simulink model "HybridControllerD2D2sim"  (R2019a)
settings: Solver=FixedStepDiscrete  StartTime=0.0  StopTime=inf  FixedStep=controlPeriod  RelTol=1e-3
PreLoadFcn:
  | initializeSimulation
  | initializeSCRAMNetGT
values from neighbouring files (symbols this model uses):
  controlPeriod = 1/1024    (= 0.0009765625)    [initializeSimulation.m]
undefined symbols (not defined in the file or in its folder): HybridCtrlParameters
libraries: simulink x4, HybridSimLib x1, slrtlib x1
settings Model: ExtModeArmWhenConnect=off  Creator=Andreas Schellenberg  LastModifiedBy=Andreas
settings DataIOCC: SaveFormat=Array  SaveOutput=off  SignalLogging=off  SaveTime=off  ReturnWorkspaceOutputs=off  SignalLoggingName=sigsOut
settings OptimizationCC: BlockReduction=off  OptimizeBlockIOStorage=off  BufferReuse=off  GlobalBufferReuse=off  ExpressionFolding=off  ExpressionDepthLimit=2147483647  LocalBlockOutputs=off  InitFltsAndDblsToZero=on  EfficientFloat2IntCast=on  LifeSpan=inf  SimCompilerOptimization=on  OptimizeDataStoreBuffers=off  BusAssignmentInplaceUpdate=off
settings DebuggingCC: SaveWithParameterizedLinksMsg=none  CheckSSInitialOutputMsg=off  UnderspecifiedInitializationDetection=Classic  StateNameClashWarn=warning  SFUnexpectedBacktrackingDiag=warning  SFNoUnconditionalDefaultTransitionDiag=warning  SFExecutionAtInitializationDiag=none  ArithmeticOperatorsInVariantConditions=warning
settings HardwareCC: ProdBitPerPointer=32  ProdBitPerSizeT=32  ProdBitPerPtrDiffT=32  ProdLargestAtomicFloat=None  ProdWordSize=32  ProdLongLongMode=on  ProdHWDeviceType=Generic->32-bit x86 compatible  TargetIntDivRoundTo=Zero  TargetEndianess=LittleEndian  TargetHWDeviceType=Intel->x86/Pentium
settings ModelReferenceCC: PropagateSignalLabelsOutOfModel=off
settings SFSimCC: SimCustomHeaderCode="#include \"PredictorCorrector.h\""  SimUserSources=PredictorCorrector.c  SimUserIncludeDirs="\"C:\\Program Files\\OpenFresco\\SourceCode\\SRC\\experimentalControl\\Simulink\\HybridSimToolbox\""  SimUseLocalCustomCode=off  SimParseCustomCode=off
settings RTWCC: SystemTargetFile=slrt.tlc  TemplateMakefile=slrt_default_tmf  Description=Simulink Real-Time  RTWUseLocalCustomCode=off  CustomHeaderCode="#include \"PredictorCorrector.h\""  CustomInclude="\"C:\\Program Files\\OpenFresco\\SourceCode\\SRC\\experimentalControl\\Simulink\\HybridSimToolbox\""  CustomSource=PredictorCorrector.c  CodeExecutionProfiling=on  RTWCompilerOptimization=on
settings CodeAppCC: StateflowObjectComments=on
settings SimulinkRealTimeCC: TargetFcnLib=ansi_tfl_tmw.mat  GeneratePreprocessorConditionals=Disable all  PreserveStateflowLocalDataDimensions=off
settings ConfigComp: CovMetricSettings=dw  CovHtmlReporting=on  CovSaveCumulativeToWorkspaceVar=on  CovSaveSingleToWorkspaceVar=on  CovExternalEMLEnable=off  CovSFcnEnable=off

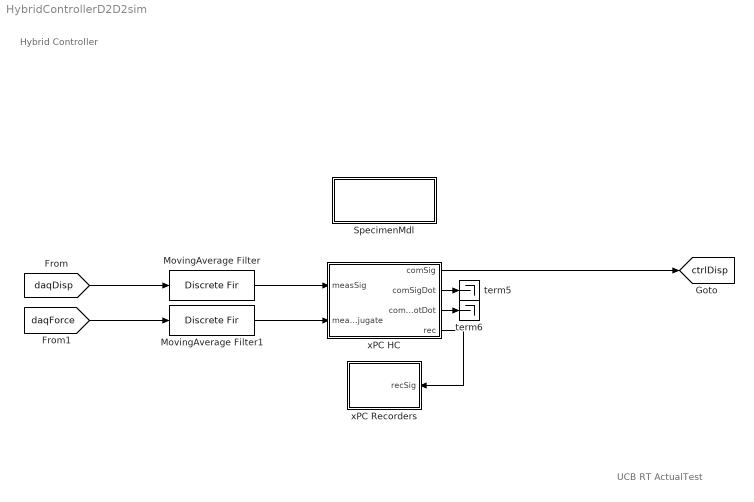
== system HybridControllerD2D2sim ==
  note: Hybrid Controller
  note: UCB RT ActualTest
  MovingAverage Filter : DiscreteFir  Coefficients=1/numSample*ones(1,numSample)  mask(Moving Average Filter){numSample=1}
      mask prompts: numSample "Number of Samples: numSample"
      mask help:
      | Moving average filter by using discrete FIR filter.
      | Set numSample = 1 for no filtering.
      mask Display: fprintf('MovingAverage\nFilter')
  MovingAverage Filter1 : DiscreteFir  Coefficients=1/numSample*ones(1,numSample)  mask(Moving Average Filter){numSample=1}
      mask prompts: numSample "Number of Samples: numSample"
      mask help:
      | Moving average filter by using discrete FIR filter.
      | Set numSample = 1 for no filtering.
      mask Display: fprintf('MovingAverage\nFilter')
  SpecimenMdl : Subsystem
      mask Display: fprintf('Test\nSpecimen');
  term5 : Terminator
  term6 : Terminator
  xPC HC : Subsystem  mask(Hybrid Controller: D2/D2){hcp=HybridCtrlParameters, node=struct([])}
      mask prompts: hcp "Hybrid control parameter structure"; node "SCRAMNet node structure"
      mask help: Hybrid Controller using C0-continuous quadratic Lagrange interpolation for prediction and correction
      mask init:
      | if isfield(hcp,'nDOF')
      |     nDOF = hcp.nDOF;
      | else
      |     nDOF = 1;
      | end
      | if isfield(hcp,'upFact')
      |     upFact = hcp.upFact;
      | else
      |     upFact = 1;
      | end
      | if isfield(hcp,'iDelay')
      |     iDelay = hcp.iDelay;
      | else
      |     iDelay = zeros(nDOF);
      | end
      | dtInt = hcp.dtInt;
      | dtSim = hcp.dtSim;
      | dtCon = hcp.dtCon;
      | N = hcp.N;
      mask Display: disp('xPC Target\nHybrid Controller\n(D2/D2)')
  xPC Recorders : Subsystem  mask{nDOF=HybridCtrlParameters.nDOF}
      mask prompts: nDOF "Number of DOF: nDOF"
  tag scope: ctrlDisp=global
  wires:
  [daqDisp] -> MovingAverage Filter/1
  xPC HC/1(comSig) -> [ctrlDisp]
  [daqForce] -> MovingAverage Filter1/1
  xPC HC/2(comSigDot) -> term5/1
  xPC HC/3(comSigDotDot) -> term6/1
  xPC HC/4(rec) -> xPC Recorders/1(recSig)
  MovingAverage Filter/1 -> xPC HC/1(measSig)
  MovingAverage Filter1/1 -> xPC HC/2(measSigConjugate)

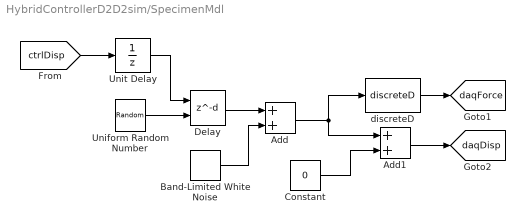
== system HybridControllerD2D2sim/SpecimenMdl ==
  Add : Sum
  Add1 : Sum
  Band-Limited White Noise : simulink/Sources/Band-Limited White Noise  Cov=1e-7  Ts=controlPeriod  seed=[23341]
  Constant : Constant  Value=0
  Delay : Delay  DelayLengthSource=Input port  DelayLengthUpperLimit=20
      settings: InputPortMap=u0,p1
  Uniform Random Number : UniformRandomNumber  Minimum=0  Maximum=2  SampleTime=controlPeriod
  Unit Delay : UnitDelay  SampleTime=-1  HasFrameUpgradeWarning=on
  discreteD : HybridSimLib/Material Models/discreteD  k=2.8  fy=1.5  alpha=0.01  beta=0.5  gamma=0.5  n=2  dt=controlPeriod
      settings: SourceProductName=Hybrid Simulation
  tag scope: daqDisp=global, daqForce=global
  wires:
  discreteD/1 -> [daqForce]
  Add/1 -> Add1/1, discreteD/1
  Delay/1 -> Add/1
  Band-Limited White Noise/1 -> Add/2
  Uniform Random Number/1 -> Delay/2
  [ctrlDisp] -> Unit Delay/1
  Unit Delay/1 -> Delay/1
  Add1/1 -> [daqDisp]
  Constant/1 -> Add1/2

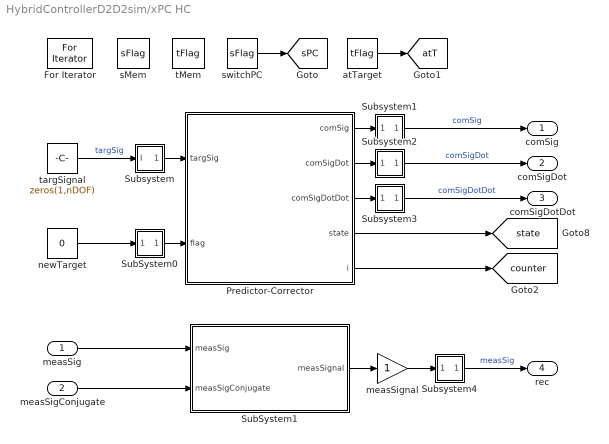
== system HybridControllerD2D2sim/xPC HC ==
  measSig : Inport
  measSigConjugate : Inport  Port=2
  For Iterator : ForIterator  IterationLimit=upFact  ShowIterationPort=off
  Predictor-Corrector : Stateflow chart  TreatAsAtomicUnit=on
  SubSystem0 : Subsystem
      mask Display: disp('I/O')
  SubSystem1 : Subsystem
  Subsystem : Subsystem
      mask Display: disp('I/O')
  Subsystem1 : Subsystem
      mask Display: disp('I/O')
  Subsystem2 : Subsystem
      mask Display: disp('I/O')
  Subsystem3 : Subsystem
      mask Display: disp('I/O')
  Subsystem4 : Subsystem
      mask Display: disp('I/O')
  atTarget : DataStoreRead  DataStoreName=tFlag
  measSignal : Gain  OutDataTypeStr=double
  newTarget : Constant  Value=0  OutDataTypeStr=int32  SampleTime=-1
  sMem : DataStoreMemory  DataStoreName=sFlag  ShowAdditionalParam=off  OutDataTypeStr=int32
  switchPC : DataStoreRead  DataStoreName=sFlag
  tMem : DataStoreMemory  DataStoreName=tFlag  ShowAdditionalParam=off  OutDataTypeStr=int32
  targSignal : Constant  Value=zeros(1,nDOF)  OutDataTypeStr=double  SampleTime=-1
  comSig : Outport
  comSigDot : Outport  Port=2
  comSigDotDot : Outport  Port=3
  rec : Outport  Port=4
  tag scope: atT=global, counter=global, sPC=global, state=global
  wires:
  measSignal/1 -> Subsystem4/1(measSig)
  SubSystem1/1(measSignal) -> measSignal/1
  Predictor-Corrector/5(i) -> [counter]
  SubSystem0/1(Out) -> Predictor-Corrector/2(flag)
  switchPC/1 -> [sPC]
  atTarget/1 -> [atT]
  targSignal/1 -> Subsystem/1(I)  "targSig"
  Subsystem/1(O) -> Predictor-Corrector/1(targSig)
  measSig/1 -> SubSystem1/1(measSig)
  measSigConjugate/1 -> SubSystem1/2(measSigConjugate)
  Predictor-Corrector/1(comSig) -> Subsystem1/1(In)
  Predictor-Corrector/2(comSigDot) -> Subsystem2/1(In)
  Predictor-Corrector/3(comSigDotDot) -> Subsystem3/1(In)
  newTarget/1 -> SubSystem0/1(In)
  Predictor-Corrector/4(state) -> [state]
  Subsystem2/1(Out) -> comSigDot/1  "comSigDot"
  Subsystem3/1(Out) -> comSigDotDot/1  "comSigDotDot"
  Subsystem1/1(Out) -> comSig/1  "comSig"
  Subsystem4/1(Out1) -> rec/1  "measSig"

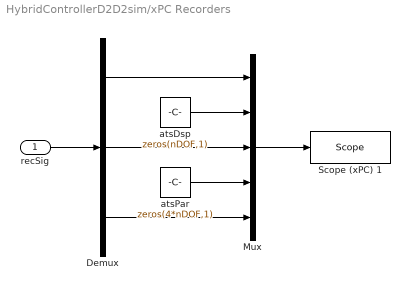
== system HybridControllerD2D2sim/xPC Recorders ==
  recSig : Inport
  Demux : Demux  Outputs=[(4*nDOF) (4*nDOF) 5]
  Mux : Mux  Inputs=5
  Scope (xPC) 1 : slrtlib/Displays and Logging/Scope   scopeno=1  scopetype=File  autostart=on  viewmode=Numerical  formatstr='%15.6f'  grid=on  ylimits=[-4,4]  nosamples=60*1024  noprepostsamples=0  interleave=1  triggermode=FreeRun  triggersignal=1  trigsignalfromport=off  triggerlevel=0.0  triggerslope=Either  triggerscope=1  triggersample=0  filename=H:\xpcRec.dat  mode=Lazy  writesize=512  autorestart=on  dynamicfilemode=off  maxwritefilesize=512*1024^2
  atsDsp : Constant  Value=zeros(nDOF,1)
  atsPar : Constant  Value=zeros(4*nDOF,1)
  wires:
  recSig/1 -> Demux/1
  atsDsp/1 -> Mux/2
  atsPar/1 -> Mux/4
  Demux/1 -> Mux/1
  Demux/2 -> Mux/3
  Mux/1 -> Scope (xPC) 1/1
  Demux/3 -> Mux/5

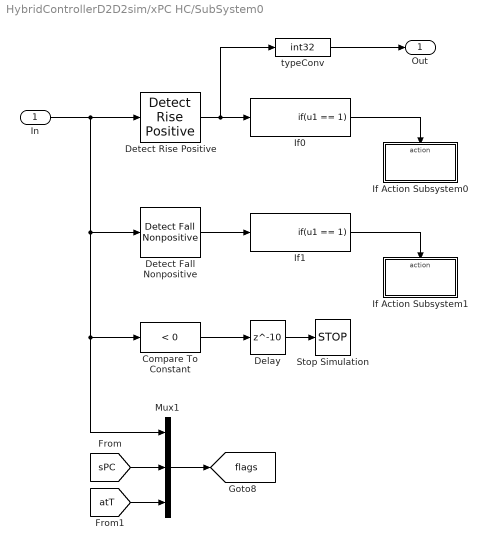
== system HybridControllerD2D2sim/xPC HC/SubSystem0 ==
  In : Inport
  Compare To Constant : simulink/Logic and Bit Operations/Compare To Constant  relop=<  const=0  OutDataTypeStr=boolean
  Delay : Delay  DelayLength=10
  Detect Fall Nonpositive : simulink/Logic and Bit Operations/Detect Fall Nonpositive  vinit=0  OutDataTypeStr=uint8
      settings: SourceProductName=Simulink  SourceProductBaseCode=SL
  Detect Rise Positive : simulink/Logic and Bit Operations/Detect Rise Positive  vinit=0  OutDataTypeStr=uint8
  If Action Subsystem0 : Subsystem  TreatAsAtomicUnit=on
  If Action Subsystem1 : Subsystem  TreatAsAtomicUnit=on
  If0 : If  IfExpression=u1 == 1  ShowElse=off
  If1 : If  IfExpression=u1 == 1  ShowElse=off
  Mux1 : Mux  Inputs=3
  Stop Simulation : Stop
  typeConv : DataTypeConversion  OutDataTypeStr=int32  SaturateOnIntegerOverflow=on  RndMeth=Zero
  Out : Outport
  tag scope: flags=global
  wires:
  Detect Rise Positive/1 -> If0/1, typeConv/1
  Detect Fall Nonpositive/1 -> If1/1
  If1/1 -> If Action Subsystem1/Action
  If0/1 -> If Action Subsystem0/Action
  typeConv/1 -> Out/1
  Mux1/1 -> [flags]
  [sPC] -> Mux1/2
  [atT] -> Mux1/3
  In/1 -> Detect Rise Positive/1, Detect Fall Nonpositive/1, Compare To Constant/1, Mux1/1
  Compare To Constant/1 -> Delay/1
  Delay/1 -> Stop Simulation/1

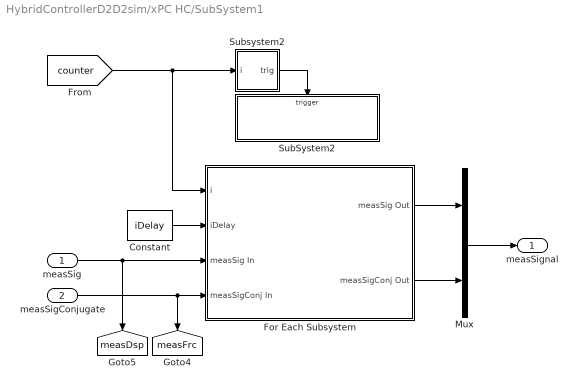
== system HybridControllerD2D2sim/xPC HC/SubSystem1 ==
  measSig : Inport
  measSigConjugate : Inport  Port=2
  Constant : Constant  Value=iDelay
  For Each Subsystem : Subsystem  TreatAsAtomicUnit=on
  Mux : Mux  Inputs=2
  SubSystem2 : Subsystem  TreatAsAtomicUnit=on
  Subsystem2 : Subsystem
  measSignal : Outport
  tag scope: measDsp=global, measFrc=global
  wires:
  Subsystem2/1(trig) -> SubSystem2/Trigger
  [counter] -> Subsystem2/1(i), For Each Subsystem/1(i)
  Constant/1 -> For Each Subsystem/2(iDelay)
  measSig/1 -> For Each Subsystem/3(measSig In), [measDsp]
  measSigConjugate/1 -> For Each Subsystem/4(measSigConj In), [measFrc]
  For Each Subsystem/1(measSig Out) -> Mux/1
  For Each Subsystem/2(measSigConj Out) -> Mux/2
  Mux/1 -> measSignal/1

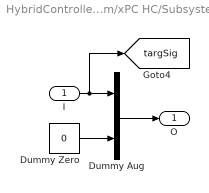
== system HybridControllerD2D2sim/xPC HC/Subsystem ==
  I : Inport  PortDimensions=nDOF
  Dummy Aug : Mux  Inputs=[nDOF 1]
  Dummy Zero : Constant  Value=0  OutDataTypeStr=double  SampleTime=-1
  O : Outport  PortDimensions=nDOF+1
  tag scope: targSig=global
  wires:
  Dummy Zero/1 -> Dummy Aug/2
  I/1 -> Dummy Aug/1, [targSig]
  Dummy Aug/1 -> O/1

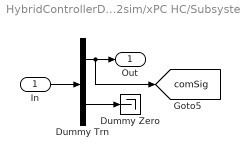
== system HybridControllerD2D2sim/xPC HC/Subsystem1 ==
  In : Inport  PortDimensions=nDOF+1
  Dummy Trn : Demux  Outputs=[nDOF 1]
  Dummy Zero : Terminator
  Out : Outport  PortDimensions=nDOF
  tag scope: comSig=global
  wires:
  Dummy Trn/2 -> Dummy Zero/1
  Dummy Trn/1 -> Out/1, [comSig]
  In/1 -> Dummy Trn/1

== system HybridControllerD2D2sim/xPC HC/Subsystem2 ==
  In : Inport  PortDimensions=nDOF+1
  Dummy Trn : Demux  Outputs=[nDOF 1]
  Dummy Zero : Terminator
  Out : Outport  PortDimensions=nDOF
  tag scope: comSigDot=global
  wires:
  Dummy Trn/2 -> Dummy Zero/1
  Dummy Trn/1 -> Out/1, [comSigDot]
  In/1 -> Dummy Trn/1

== system HybridControllerD2D2sim/xPC HC/Subsystem3 ==
  In : Inport  PortDimensions=nDOF+1
  Dummy Trn : Demux  Outputs=[nDOF 1]
  Dummy Zero : Terminator
  Out : Outport  PortDimensions=nDOF
  tag scope: comSigDotDot=global
  wires:
  Dummy Trn/2 -> Dummy Zero/1
  Dummy Trn/1 -> Out/1, [comSigDotDot]
  In/1 -> Dummy Trn/1

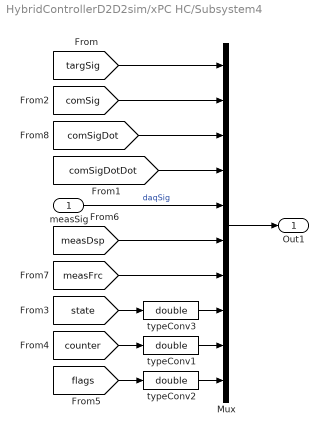
== system HybridControllerD2D2sim/xPC HC/Subsystem4 ==
  measSig : Inport
  Mux : Mux  Inputs=10
  typeConv1 : DataTypeConversion  OutDataTypeStr=double  SaturateOnIntegerOverflow=on  RndMeth=Zero
  typeConv2 : DataTypeConversion  OutDataTypeStr=double  SaturateOnIntegerOverflow=on  RndMeth=Zero
  typeConv3 : DataTypeConversion  OutDataTypeStr=double  SaturateOnIntegerOverflow=on  RndMeth=Zero
  Out1 : Outport
  wires:
  measSig/1 -> Mux/5  "daqSig"
  [flags] -> typeConv2/1
  [counter] -> typeConv1/1
  [state] -> typeConv3/1
  typeConv3/1 -> Mux/8
  typeConv1/1 -> Mux/9
  typeConv2/1 -> Mux/10
  [measFrc] -> Mux/7
  [measDsp] -> Mux/6
  [comSigDotDot] -> Mux/4
  [comSigDot] -> Mux/3
  [comSig] -> Mux/2
  [targSig] -> Mux/1
  Mux/1 -> Out1/1

== system HybridControllerD2D2sim/xPC HC/SubSystem0/If Action Subsystem0 ==
  Action Port : ActionPort  PropagateVarSize=During execution  ActionPortLabel=if(u1 == 1)
  Data Store Write0 : DataStoreWrite  DataStoreName=sFlag
  Data Store Write1 : DataStoreWrite  DataStoreName=tFlag
  atTargetFlag : Constant  Value=0  OutDataTypeStr=int32  SampleTime=-1
  switchFlag : Constant  OutDataTypeStr=int32  SampleTime=-1
  wires:
  atTargetFlag/1 -> Data Store Write1/1
  switchFlag/1 -> Data Store Write0/1

== system HybridControllerD2D2sim/xPC HC/SubSystem0/If Action Subsystem1 ==
  Action Port : ActionPort  PropagateVarSize=During execution  ActionPortLabel=if(u1 == 1)
  Data Store Write0 : DataStoreWrite  DataStoreName=sFlag
  switchFlag : Constant  Value=0  OutDataTypeStr=int32  SampleTime=-1
  wires:
  switchFlag/1 -> Data Store Write0/1

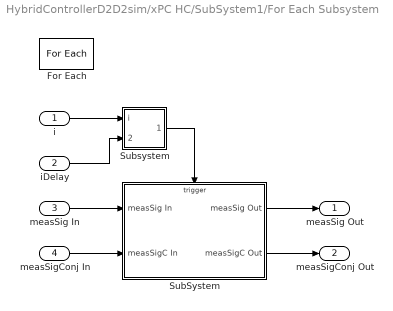
== system HybridControllerD2D2sim/xPC HC/SubSystem1/For Each Subsystem ==
  i : Inport
  iDelay : Inport  Port=2  Partition=on  PartitionDimension=1  PartitionWidth=1  PartitionOffset=0
  measSig In : Inport  Port=3  Partition=on  PartitionDimension=1  PartitionWidth=1  PartitionOffset=0
  measSigConj In : Inport  Port=4  Partition=on  PartitionDimension=1  PartitionWidth=1  PartitionOffset=0
  For Each : ForEach  DisableCoverage=on  IndexMode=One-based
  SubSystem : Subsystem  TreatAsAtomicUnit=on
  Subsystem : Subsystem
  measSig Out : Outport  ConcatenationDimension=1
  measSigConj Out : Outport  Port=2  ConcatenationDimension=1
  wires:
  Subsystem/1(trig) -> SubSystem/Trigger
  measSig In/1 -> SubSystem/1(measSig In)
  measSigConj In/1 -> SubSystem/2(measSigC In)
  SubSystem/1(measSig Out) -> measSig Out/1
  SubSystem/2(measSigC Out) -> measSigConj Out/1
  iDelay/1 -> Subsystem/2(iDelay)
  i/1 -> Subsystem/1(i)

== system HybridControllerD2D2sim/xPC HC/SubSystem1/SubSystem2 ==
  Trigger : TriggerPort  VariantControl=(inherit)
  Data Store Write : DataStoreWrite  DataStoreName=tFlag
  atTargetFlag : Constant  OutDataTypeStr=int32  SampleTime=-1
  wires:
  atTargetFlag/1 -> Data Store Write/1

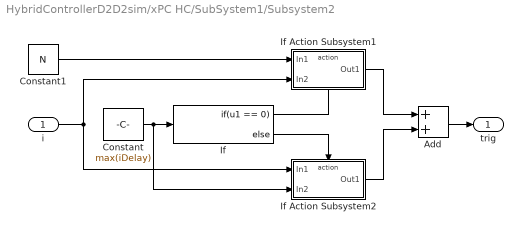
== system HybridControllerD2D2sim/xPC HC/SubSystem1/Subsystem2 ==
  i : Inport
  Add : Sum
  Constant : Constant  Value=max(iDelay)
  Constant1 : Constant  Value=N
  If : If  IfExpression=u1 == 0
  If Action Subsystem1 : Subsystem  TreatAsAtomicUnit=on
  If Action Subsystem2 : Subsystem  TreatAsAtomicUnit=on
  trig : Outport
  wires:
  Constant/1 -> If/1, If Action Subsystem2/2(In2)
  If/1 -> If Action Subsystem1/Action
  If/2 -> If Action Subsystem2/Action
  If Action Subsystem1/1(Out1) -> Add/1
  If Action Subsystem2/1(Out1) -> Add/2
  Add/1 -> trig/1
  i/1 -> If Action Subsystem1/2(In2), If Action Subsystem2/1(In1)
  Constant1/1 -> If Action Subsystem1/1(In1)

== system HybridControllerD2D2sim/xPC HC/SubSystem1/For Each Subsystem/SubSystem ==
  measSig In : Inport
  measSigC In : Inport  Port=2
  Trigger : TriggerPort  VariantControl=(inherit)
  measSig Out : Outport  InitialOutput=[0]
  measSigC Out : Outport  Port=2  InitialOutput=[0]
  wires:
  measSigC In/1 -> measSigC Out/1
  measSig In/1 -> measSig Out/1

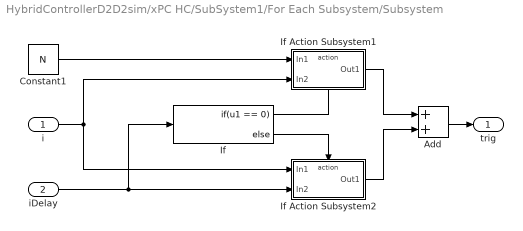
== system HybridControllerD2D2sim/xPC HC/SubSystem1/For Each Subsystem/Subsystem ==
  i : Inport
  iDelay : Inport  Port=2
  Add : Sum
  Constant1 : Constant  Value=N
  If : If  IfExpression=u1 == 0
  If Action Subsystem1 : Subsystem  TreatAsAtomicUnit=on
  If Action Subsystem2 : Subsystem  TreatAsAtomicUnit=on
  trig : Outport
  wires:
  iDelay/1 -> If/1, If Action Subsystem2/2(In2)
  If/1 -> If Action Subsystem1/Action
  If/2 -> If Action Subsystem2/Action
  If Action Subsystem1/1(Out1) -> Add/1
  If Action Subsystem2/1(Out1) -> Add/2
  Add/1 -> trig/1
  i/1 -> If Action Subsystem1/2(In2), If Action Subsystem2/1(In1)
  Constant1/1 -> If Action Subsystem1/1(In1)

== system HybridControllerD2D2sim/xPC HC/SubSystem1/Subsystem2/If Action Subsystem1 ==
  In1 : Inport
  In2 : Inport  Port=2
  Action Port : ActionPort  ActionPortLabel=if(u1 == 0)
  Relational Operator : RelationalOperator  Operator===  OutDataTypeStr=boolean  RndMeth=Nearest
  Out1 : Outport  InitialOutput=0
  wires:
  Relational Operator/1 -> Out1/1
  In1/1 -> Relational Operator/1
  In2/1 -> Relational Operator/2

== system HybridControllerD2D2sim/xPC HC/SubSystem1/Subsystem2/If Action Subsystem2 ==
  In1 : Inport
  In2 : Inport  Port=2
  Action Port : ActionPort  ActionPortLabel=else
  Relational Operator : RelationalOperator  Operator===  OutDataTypeStr=boolean  RndMeth=Nearest
  Out1 : Outport  InitialOutput=0
  wires:
  Relational Operator/1 -> Out1/1
  In1/1 -> Relational Operator/1
  In2/1 -> Relational Operator/2

== system HybridControllerD2D2sim/xPC HC/SubSystem1/For Each Subsystem/Subsystem/If Action Subsystem1 ==
  In1 : Inport
  In2 : Inport  Port=2
  Action Port : ActionPort  ActionPortLabel=if(u1 == 0)
  Relational Operator : RelationalOperator  Operator===  OutDataTypeStr=boolean  RndMeth=Nearest
  Out1 : Outport  InitialOutput=0
  wires:
  Relational Operator/1 -> Out1/1
  In1/1 -> Relational Operator/1
  In2/1 -> Relational Operator/2

== system HybridControllerD2D2sim/xPC HC/SubSystem1/For Each Subsystem/Subsystem/If Action Subsystem2 ==
  In1 : Inport
  In2 : Inport  Port=2
  Action Port : ActionPort  ActionPortLabel=else
  Relational Operator : RelationalOperator  Operator===  OutDataTypeStr=boolean  RndMeth=Nearest
  Out1 : Outport  InitialOutput=0
  wires:
  Relational Operator/1 -> Out1/1
  In1/1 -> Relational Operator/1
  In2/1 -> Relational Operator/2

== stateflow chart HybridControllerD2D2sim/xPC HC/Predictor-Corrector ==
  state HybridController [parallel]
    settings: executionOrder=1
    state Initialize
      en:
      state = -1;
      i = 0; iSD = 0; diSD = 1;
      initData(nDOF,dtCon,dtSim,dtInt);
      state GetSetpoint
        en:
        setData(targSig);
        setSig(comSig,targSig);
        zeroSig(comSigDot);
        zeroSig(comSigDotDot);
        du:
        i = 0;
      (default) -> GetSetpoint
      GetSetpoint -> GetSetpoint : [after(dtCon,sec)]
          | {i=N}
    state Correct
      en:
      state = 0;
      setCurSig(comSig,i/N);
      setNewSig(targSig);
      en, du:
      di = min(max(diSD+1/(0.1*N)*(i-iSD),0.001),1.0);
      i = min(i+di,N);
      correctD2(comSig,i/N);
      correctV2(comSigDot,i/N);
      correctA2(comSigDotDot,i/N);
    state Predict
      en:
      state = 1;
      setCurSig(comSig,1.0);
      i = 1; iSD = 0; diSD = 1;
      du:
      i++;
      en, du:
      predictD2(comSig,i/N);
      predictV2(comSigDot,i/N);
      predictA2(comSigDotDot,i/N);
    state AutoSlowDown
      en:
      state = 2;
      en, du:
      diSD = 9-i/(0.1*N); i += diSD; iSD = i;
      predictD2(comSig,i/N);
      predictV2(comSigDot,i/N);
      predictA2(comSigDotDot,i/N);
    Correct -> Predict [order 1] : [flag==0 && i==N]
    (default) -> Initialize
    Initialize -> Correct : [flag==1]
        | {i=0}
    Predict -> Correct [order 2] : [flag==1]
    Predict -> AutoSlowDown [order 1] : [flag==0 && i>=0.8*N]
    AutoSlowDown -> Correct : [flag==1]
    Correct -> Correct [order 2] : [flag==1]
        | {i=0; iSD=0; diSD=1}
  data: targSig input double size=nDOF+1; flag input int32; comSig output double size=nDOF+1; comSigDot output double size=nDOF+1; comSigDotDot output double size=nDOF+1; state output int32; i output double; N parameter int32; nDOF parameter int32; di local double; diSD local double; iSD local double; dtCon parameter double; dtSim parameter double; dtInt parameter double
